simulink model "16-QAM"  (R2022b)
settings: Solver=VariableStepAuto  StartTime=0.0  StopTime=10.0  RelTol=1e-3
undefined symbols (not defined in the file): QAM
libraries: dspsrcs4 x4, dspstat3 x3, simulink x2, dsparch4 x2, commsink2 x2, commutil2 x2, commdigbbndam3 x2, commchan3 x1, commrandsrc3 x1
settings Model: Creator=metal  LastModifiedBy=metal

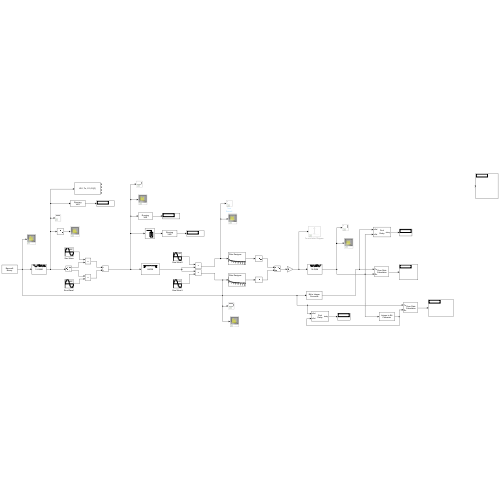
[thumbnail: Simulink's stored preview of the top-level diagram]
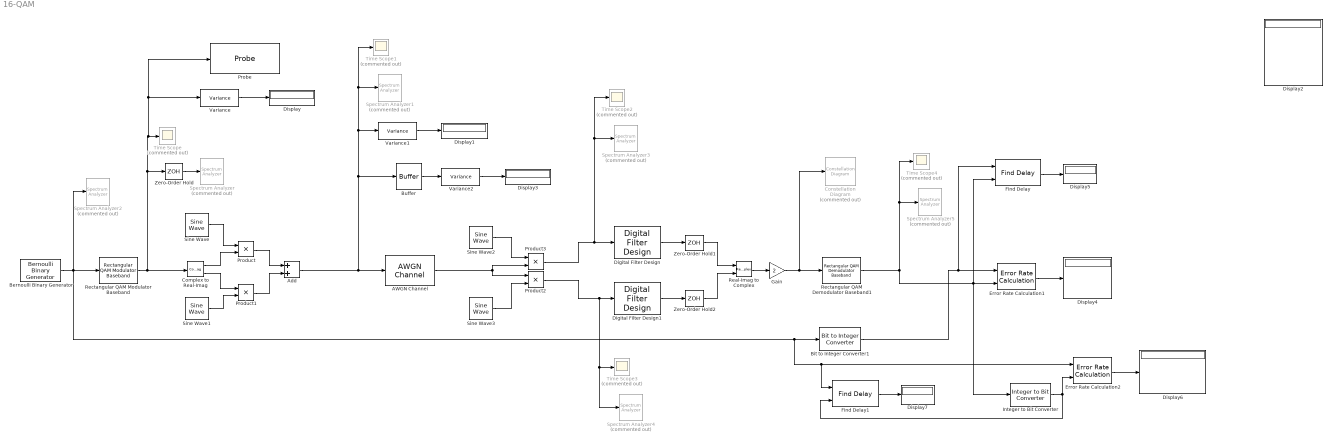
== system 16-QAM ==
  AWGN Channel : commchan3/AWGN Channel  InputProcessing=Columns as channels (frame based)  seed=67  noiseMode="Signal to noise ratio  (Eb/No)"  EbNodB=20  EsNodB=10  SNRdB=10  bitsPerSym=4  Ps=1/2  Tsym=1/(1e6/4)  variance=1
  Add : Sum
  Bernoulli Binary Generator : commrandsrc3/Bernoulli Binary Generator  ProbabilityOfZero=0.5  SeedSource=Parameter  Seed=41  SampleTime=1/1e6  SamplesPerFrame=4  OutputDataType=double  SimulateUsing=Interpreted execution
  Bit to Integer Converter1 : simulink/Logic and Bit Operations/Bit to Integer Converter  nbits=4  bitOrder=MSB first  signedOutputValues=Unsigned  outDtype=Inherit via internal rule  outDtypeSigned=Inherit via internal rule
  Buffer : Buffer  OutputFrames=off
  Complex to Real-Imag : ComplexToRealImag
  Constellation Diagram : ConstellationDiagram  Commented=on  WindowPosition=[162.000000,94.000000,864.000000,600.000000,]  ScopeFrameLocation=window  SymbolsToDisplaySource=Property  SymbolsToDisplay=1000  ReferenceConstellation=16-QAM  XLimits=[-1.39,1.39]  YLimits=[-1.38,1.38]  EnableMeasurements=on  MeasurementInterval=All displays
  Digital Filter Design : dsparch4/Digital Filter Design  mwdsp_browser_bugfix_var=off
  Digital Filter Design1 : dsparch4/Digital Filter Design  mwdsp_browser_bugfix_var=off
  Display{,1..7} (8 alike) : Display
      Display2 settings: Format=decimal (Stored Integer)
      Display4 settings: Format=decimal (Stored Integer)
      Display5 settings: Format=decimal (Stored Integer)
      Display6 settings: Format=decimal (Stored Integer)
      Display7 settings: Format=decimal (Stored Integer)
  Error Rate Calculation1 : commsink2/Error Rate Calculation  N=1  st_delay=0  cp_mode=Entire frame  subframe=[]  PMode=Port  WsName=ErrorVec  RsMode2=off  stop=off  numErr=100  maxBits=1e6
  Error Rate Calculation2 : commsink2/Error Rate Calculation  N=4  st_delay=0  cp_mode=Entire frame  subframe=[]  PMode=Port  WsName=ErrorVec  RsMode2=off  stop=off  numErr=100  maxBits=1e6
  Find Delay : commutil2/Find Delay  corrLength=200  chgSigOP=off  stopUpdate=off  numConstDelay=3
  Find Delay1 : commutil2/Find Delay  corrLength=200  chgSigOP=off  stopUpdate=off  numConstDelay=3
  Gain : Gain  Gain=2
  Integer to Bit Converter : simulink/Logic and Bit Operations/Integer to Bit Converter  nbits=4  signedInputValues=Unsigned  bitOrder=MSB first  outDtype=Inherit via internal rule
  Probe : Probe  ProbeSignalDimensions=on
  Product{,1..3} (4 alike) : Product
  Real-Imag to Complex : RealImagToComplex
  Rectangular QAM Demodulator Baseband1 : commdigbbndam3/Rectangular QAM Demodulator Baseband  M=16  OutType=Integer  DecType=Hard decision  VarSource=Dialog  Variance=1  Dec=Gray  Mapping=[0:15]  PowType=Average Power  MinDist=2  AvgPow=1  PeakPow=1  Ph=0  outDtype1=Inherit via internal rule  outDtype2=Inherit via internal rule  derotateFactorWordLen=16  derotateFactorDataTypeStr=Inherit: Same word length as input  derotateFactorLastDataTypeStr=Inherit: Same word length as input  denormFactorWordLen=16  denormFactorDataTypeStr=Inherit: Same word length as input  denormFactorLastDataTypeStr=Inherit: Same word length as input  prodOutWordLen=32  prodOutOverflowMode=Wrap  prodOutRoundingMode=Floor  prodOutOvFlMode=off  prodOutOvFlModeLastStrValue=off  sumWordLen=32
  Rectangular QAM Modulator Baseband : commdigbbndam3/Rectangular QAM Modulator Baseband  M=16  InType=Bit  Enc=Gray  Mapping=[0:15]  PowType=Average Power  MinDist=2  AvgPow=1  PeakPow=1  Ph=0  outDtype=double  outWordLen=16  outUDDataType=sfix(16)  outFracLenMode=Best precision  outFracLen=15  outDataTypeStr=double  outLastDataTypeStr=double
  Sine Wave : dspsrcs4/Sine Wave  Amplitude=1  Frequency=10e6  Phase=pi/2  SampleMode=Discrete  OutComplex=Real  CompMethod=Trigonometric fcn  TableSize=Speed  SampleTime=1/100e6  SamplesPerFrame=1  ResetState=Restart at time zero  OutputFrames=off  dataType=double  wordLen=16  udDataType=sfix(16)  fracBitsMode=Best precision  numFracBits=15  OutDataTypeStr=double  LastOutDataTypeStr=double
  Sine Wave1 : dspsrcs4/Sine Wave  Amplitude=1  Frequency=10e6  Phase=0  SampleMode=Discrete  OutComplex=Real  CompMethod=Trigonometric fcn  TableSize=Speed  SampleTime=1/100e6  SamplesPerFrame=1  ResetState=Restart at time zero  OutputFrames=off  dataType=double  wordLen=16  udDataType=sfix(16)  fracBitsMode=Best precision  numFracBits=15  OutDataTypeStr=double  LastOutDataTypeStr=double
  Sine Wave2 : dspsrcs4/Sine Wave  Amplitude=1  Frequency=10e6  Phase=pi/2  SampleMode=Discrete  OutComplex=Real  CompMethod=Trigonometric fcn  TableSize=Speed  SampleTime=1/100e6  SamplesPerFrame=1  ResetState=Restart at time zero  OutputFrames=off  dataType=double  wordLen=16  udDataType=sfix(16)  fracBitsMode=Best precision  numFracBits=15  OutDataTypeStr=double  LastOutDataTypeStr=double
  Sine Wave3 : dspsrcs4/Sine Wave  Amplitude=1  Frequency=10e6  Phase=0  SampleMode=Discrete  OutComplex=Real  CompMethod=Trigonometric fcn  TableSize=Speed  SampleTime=1/100e6  SamplesPerFrame=1  ResetState=Restart at time zero  OutputFrames=off  dataType=double  wordLen=16  udDataType=sfix(16)  fracBitsMode=Best precision  numFracBits=15  OutDataTypeStr=double  LastOutDataTypeStr=double
  Spectrum Analyzer{,1..5} (6 alike) : SpectrumAnalyzer  Commented=on
  Time Scope{,1..4} (5 alike) : Scope  Commented=on
  Variance : dspstat3/Variance  run=on  InputProcessing=Columns as channels (frame based)  reset_popup=None  directionMode=Each column  dimension=1  roiEnable=off  roiType=Rectangles  roiPortion=Entire ROI  roiOutput=Individual statistics for each ROI  roiFlag=off  roundingMode=Floor  overflowMode=off
  Variance1 : dspstat3/Variance  run=on  InputProcessing=Columns as channels (frame based)  reset_popup=None  directionMode=Each column  dimension=1  roiEnable=off  roiType=Rectangles  roiPortion=Entire ROI  roiOutput=Individual statistics for each ROI  roiFlag=off  roundingMode=Floor  overflowMode=off
  Variance2 : dspstat3/Variance  run=on  InputProcessing=Columns as channels (frame based)  reset_popup=None  directionMode=Each column  dimension=1  roiEnable=off  roiType=Rectangles  roiPortion=Entire ROI  roiOutput=Individual statistics for each ROI  roiFlag=off  roundingMode=Floor  overflowMode=off
  Zero-Order Hold : ZeroOrderHold  SampleTime=1/1000000
  Zero-Order Hold1 : ZeroOrderHold  SampleTime=1/250e3
  Zero-Order Hold2 : ZeroOrderHold  SampleTime=1/250e3
  wires:
  Bernoulli Binary Generator/1 -> Find Delay1/1, Error Rate Calculation2/1, Bit to Integer Converter1/1, Spectrum Analyzer2/1, Rectangular QAM Modulator Baseband/1
  Complex to Real-Imag/2 -> Product1/1
  Sine Wave1/1 -> Product1/2
  Sine Wave/1 -> Product/1
  Complex to Real-Imag/1 -> Product/2
  Product/1 -> Add/1
  Product1/1 -> Add/2
  Rectangular QAM Modulator Baseband/1 -> Zero-Order Hold/1, Variance/1, Probe/1, Time Scope/1, Complex to Real-Imag/1
  Add/1 -> AWGN Channel/1, Buffer/1, Variance1/1, Time Scope1/1, Spectrum Analyzer1/1
  Zero-Order Hold/1 -> Spectrum Analyzer/1
  Variance/1 -> Display/1
  Variance1/1 -> Display1/1
  AWGN Channel/1 -> Product3/2, Product2/1
  Sine Wave2/1 -> Product3/1
  Sine Wave3/1 -> Product2/2
  Digital Filter Design/1 -> Zero-Order Hold1/1
  Digital Filter Design1/1 -> Zero-Order Hold2/1
  Zero-Order Hold1/1 -> Real-Imag to Complex/1
  Zero-Order Hold2/1 -> Real-Imag to Complex/2
  Real-Imag to Complex/1 -> Gain/1
  Gain/1 -> Constellation Diagram/1, Rectangular QAM Demodulator Baseband1/1
  Product3/1 -> Time Scope2/1, Spectrum Analyzer3/1, Digital Filter Design/1
  Product2/1 -> Digital Filter Design1/1, Spectrum Analyzer4/1, Time Scope3/1
  Rectangular QAM Demodulator Baseband1/1 -> Integer to Bit Converter/1, Error Rate Calculation1/2, Find Delay/2, Time Scope4/1, Spectrum Analyzer5/1
  Variance2/1 -> Display3/1
  Buffer/1 -> Variance2/1
  Bit to Integer Converter1/1 -> Find Delay/1, Error Rate Calculation1/1
  Error Rate Calculation1/1 -> Display4/1
  Find Delay/1 -> Display5/1
  Integer to Bit Converter/1 -> Find Delay1/2, Error Rate Calculation2/2
  Error Rate Calculation2/1 -> Display6/1
  Find Delay1/1 -> Display7/1
